simulink model "sl_MCD_sincrono"  (R2016b)
settings: Solver=VariableStepAuto  StartTime=0.0  StopTime=t_sim  RelTol=1e-3
values from neighbouring files (symbols this model uses):
  ampl_sin = 2    [pruebas_MCD.m]    (also in pruebas_modelo.m)
  freq = 0.25    [pruebas_MCD.m]    (also in pruebas_modelo.m)
  omega = in(2)    [MCD_movil.m]    (also in MCI_movil.m = jac_inv(2,:)*gen; control_linea.m = -Kd*d+Kh*err_ang; control_persecucion.m = v_ref/R; control_tray.m = Kh*(phi_ref-phi))
  omega_sat = [-0.2618 0.2618]    [prueba_persecucionPURA.m]    (also in pruebas_MCD.m; pruebas_control.m; pruebas_control_P2.m; pruebas_modelo.m)
  pos_init = [0;0;0]    [prueba_persecucionPURA.m]    (also in pruebas_MCD.m; pruebas_control.m; pruebas_control_P2.m; pruebas_modelo.m)
  sel = in(2)    [generador_tray.m]    (also in pruebas_MCD.m = input(selection); pruebas_control_P2.m = input('Que tipo de control desea probar:\n1.Control a un pun)
  tetha_d = in(1)    [MCD_movil.m]    (also in MCI_movil.m = jac_inv(1,:)*gen; pruebas_MCD.m = 5; pruebas_modelo.m = 5)
  tetha_d_sat = [-0.75 0.75]    [prueba_persecucionPURA.m]    (also in pruebas_MCD.m; pruebas_control.m; pruebas_control_P2.m; pruebas_modelo.m)
settings Model: Creator=marrcogrova  LastModifiedBy=marrcogrova

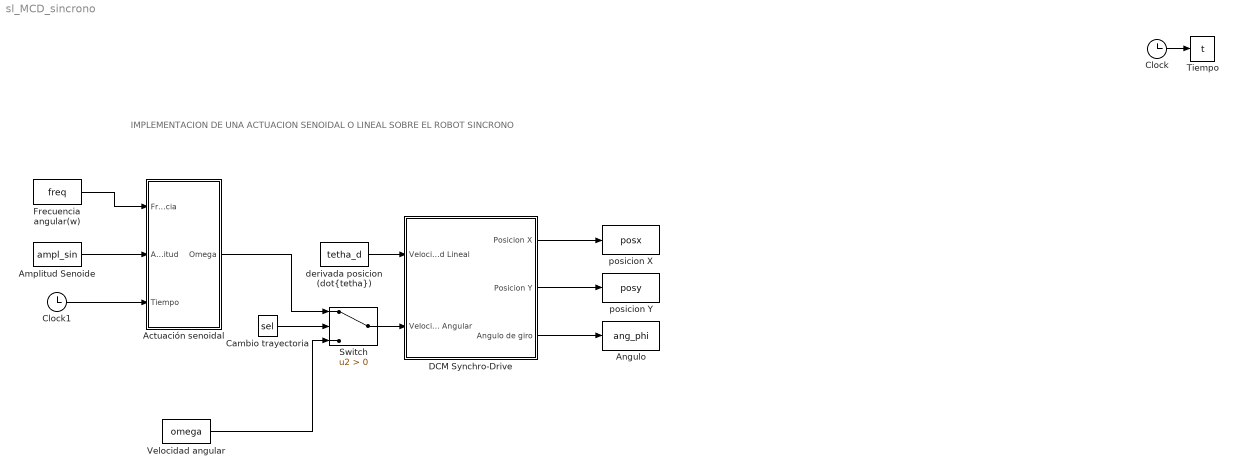
== system sl_MCD_sincrono ==
  note: IMPLEMENTACION DE UNA ACTUACION SENOIDAL
      | O LINEAL SOBRE EL ROBOT SINCRONO
  Actuación senoidal : Subsystem
  "Amplitud Senoide " : Constant  Value=ampl_sin
  Angulo : ToWorkspace  VariableName=ang_phi  SampleTime=-1
  Cambio trayectoria : Constant  Value=sel
  Clock : Clock
  Clock1 : Clock
  DCM Synchro-Drive : Subsystem
  Frecuencia angular(w) : Constant  Value=freq
  Switch : Switch  Criteria=u2 > Threshold
  Tiempo : ToWorkspace  VariableName=t  SampleTime=-1
  Velocidad angular : Constant  Value=omega
  "derivada posicion (dot{tetha})" : Constant  Value=tetha_d
  posicion X : ToWorkspace  VariableName=posx  SampleTime=-1
  posicion Y : ToWorkspace  VariableName=posy  SampleTime=-1
  wires:
  DCM Synchro-Drive/3(Angulo de giro) -> Angulo/1
  Clock/1 -> Tiempo/1
  "derivada posicion (dot{tetha})"/1 -> DCM Synchro-Drive/1(Velocidad Lineal)
  Clock1/1 -> Actuación senoidal/3(Tiempo)
  Frecuencia angular(w)/1 -> Actuación senoidal/1("Frecuencia ")
  "Amplitud Senoide "/1 -> Actuación senoidal/2("Amplitud ")
  DCM Synchro-Drive/1(Posicion X) -> posicion X/1
  DCM Synchro-Drive/2(Posicion Y) -> posicion Y/1
  Switch/1 -> DCM Synchro-Drive/2(Velocidad Angular)
  Actuación senoidal/1(Omega) -> Switch/1
  Velocidad angular/1 -> Switch/3
  Cambio trayectoria/1 -> Switch/2

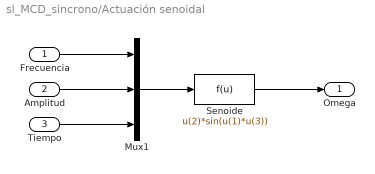
== system sl_MCD_sincrono/Actuación senoidal ==
  "Frecuencia " : Inport
  "Amplitud " : Inport  Port=2
  Tiempo : Inport  Port=3
  Mux1 : Mux  Inputs=3
  Senoide : Fcn  Expr=u(2)*sin(u(1)*u(3))
  Omega : Outport
  wires:
  Senoide/1 -> Omega/1
  "Frecuencia "/1 -> Mux1/1
  Mux1/1 -> Senoide/1
  "Amplitud "/1 -> Mux1/2
  Tiempo/1 -> Mux1/3

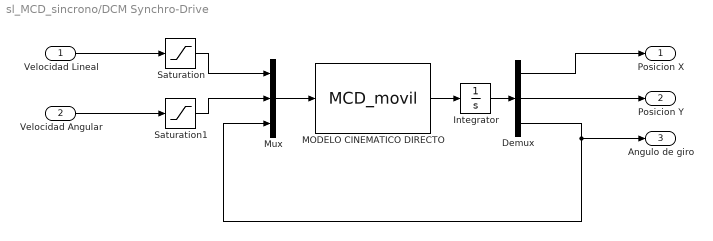
== system sl_MCD_sincrono/DCM Synchro-Drive ==
  Velocidad Lineal : Inport
  Velocidad Angular : Inport  Port=2
  Demux : Demux  Outputs=3
  Integrator : Integrator  InitialCondition=pos_init
  MODELO CINEMATICO DIRECTO : MATLABFcn  MATLABFcn=MCD_movil  OutputDimensions=3
  Mux : Mux  Inputs=3
  Saturation : Saturate  UpperLimit=tetha_d_sat(2)  LowerLimit=tetha_d_sat(1)
  Saturation1 : Saturate  UpperLimit=omega_sat(2)  LowerLimit=omega_sat(1)
  Posicion X : Outport
  Posicion Y : Outport  Port=2
  Angulo de giro : Outport  Port=3
  wires:
  Integrator/1 -> Demux/1
  Demux/3 -> Angulo de giro/1, Mux/3
  Demux/1 -> Posicion X/1
  Demux/2 -> Posicion Y/1
  Mux/1 -> MODELO CINEMATICO DIRECTO/1
  MODELO CINEMATICO DIRECTO/1 -> Integrator/1
  Velocidad Lineal/1 -> Saturation/1
  Saturation/1 -> Mux/1
  Saturation1/1 -> Mux/2
  Velocidad Angular/1 -> Saturation1/1
